simulink model "Askhsh_5"  (R2018b)
settings: Solver=VariableStepAuto  StartTime=0.0  StopTime=1  RelTol=1e-3
settings Model: Creator=mluser  LastModifiedBy=mluser
settings DataIOCC: ReturnWorkspaceOutputs=on  Refine=10
settings DebuggingCC: UnconnectedInputMsg=none  UnconnectedOutputMsg=none  UnconnectedLineMsg=none
settings ModelReferenceCC: EnableRefExpFcnMdlSchedulingChecks=off
settings RTWCC: Description=Generic Real-Time Target

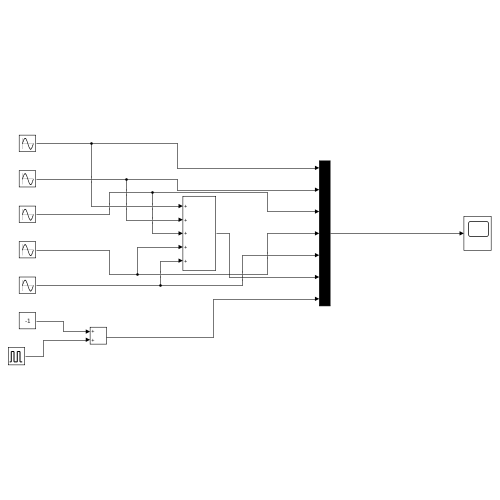
[thumbnail: Simulink's stored preview of the top-level diagram]
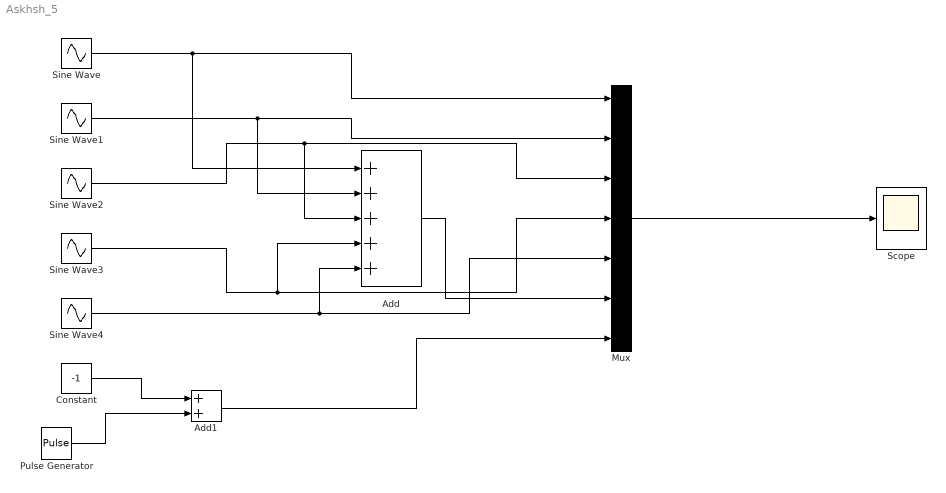
== system Askhsh_5 ==
  Add : Sum  Inputs=+++++
  Add1 : Sum
  Constant : Constant  Value=-1
  Mux : Mux  Inputs=7
  Pulse Generator : DiscretePulseGenerator  PulseType=Time based  Amplitude=2  Period=10  PulseWidth=5
  Scope : Scope
  Sine Wave : Sin  Amplitude=4/pi  Frequency=2*pi  SampleTime=0
  Sine Wave1 : Sin  Amplitude=4/(3*pi)  Frequency=6*pi  SampleTime=0
  Sine Wave2 : Sin  Amplitude=4/(5*pi)  Frequency=10*pi  SampleTime=0
  Sine Wave3 : Sin  Amplitude=4/(7*pi)  Frequency=14*pi  SampleTime=0
  Sine Wave4 : Sin  Amplitude=4/(9*pi)  Frequency=18*pi  SampleTime=0
  wires:
  Mux/1 -> Scope/1
  Constant/1 -> Add1/1
  Add1/1 -> Mux/7
  Pulse Generator/1 -> Add1/2
  Sine Wave/1 -> Add/1, Mux/1
  Sine Wave1/1 -> Add/2, Mux/2
  Sine Wave2/1 -> Add/3, Mux/3
  Sine Wave4/1 -> Add/5, Mux/5
  Add/1 -> Mux/6
  Sine Wave3/1 -> Add/4, Mux/4
